simulink model "car_model_FIXED"  (R2022b)
settings: Solver=VariableStepAuto  StartTime=0.0  StopTime=60  RelTol=1e-3
values from neighbouring files (symbols this model uses):
  ABS_MAX_TORQUE = [25 25 25 25]    [Startup.m]
  ABS_MAX_TRQ_CMD = dot(ABS_MAX_TORQUE, MOTOR_ENABLE)    [Startup.m]
  ABS_MIN_TORQUE = [0.01 0.01 0.01 0.01]    [Startup.m]
  acc_IC = 0    [Startup.m]
  ACCELERATION_MAX = 30    [Startup.m]
  ang_IC = 0    [Startup.m]
  ang_vel_IC = 0    [Startup.m]
  ax = Reference_Signals.Chassis_Acceleration_VNED.ax.Data(:)    [Simulation_Data_Parse.m]    (also in Vehicle_Sim_Parse.m)
  ay = Reference_Signals.Chassis_Acceleration_VNED.ay.Data(:)    [Simulation_Data_Parse.m]    (also in Vehicle_Sim_Parse.m)
  az = Reference_Signals.Chassis_Acceleration_VNED.az.Data(:)    [Simulation_Data_Parse.m]    (also in Vehicle_Sim_Parse.m)
  battery_current_IC = 0    [Startup.m]
  BATTERY_CURRENT_MAX = 140    [Startup.m]
  BATTERY_CURRENT_MIN = 0    [Startup.m]
  battery_FT_IC = 300    [Startup.m]
  battery_T_IC = 300    [Startup.m]
  BATTERY_TEMPERATURE_MAX = 60    [Startup.m]
  BATTERY_TEMPERATURE_MIN = 0    [Startup.m]
  battery_voltage_IC = Ns*max(Em)    [Startup.m]
  BATTERY_VOLTAGE_MAX = 340    [Startup.m]
  BATTERY_VOLTAGE_MIN = 60    [Startup.m]
  Brake_Pressure_IC = 1    [Startup.m]
  ccl_IC = 0    [Startup.m]
  CENTER_STEER_ANGLE_MAX = 130    [Startup.m]
  covarience_matrix_IC = Simulink.Parameter(eye(28)./1000)    [Startup.m]
  dcl_IC = 140    [Startup.m]
  DCL_MAX = 130    [Startup.m]
  DCL_MIN = 0    [Startup.m]
  driver_t = 0.015    [Startup.m]
  fusion_t = Simulink.Parameter(0.01)    [Startup.m]
  fusion_t_sim = fusion_t.copy    [Startup.m]
  Fz_IC = m_all*g/4    [Startup.m]
  g = 9.81    [Startup.m]
  gps_hz = 0.01    [Startup.m]
  gps_ratio = Simulink.Parameter(gps_hz / imu_hz.Value)    [Startup.m]
  imu_hz = fusion_t.copy    [Startup.m]
  location_lla_IC = Simulink.Parameter([40.437675, -86.943750, 200])    [Startup.m]
  MAG_MAX = 200    [Startup.m]
  Max_Brake_Pressure = 10^8    (= 100000000)    [Startup.m]
  Max_Driver_Input = 1    [Startup.m]
  MAX_DTHETA_DRIVER = 360    [Startup.m]
  MAX_STEERING_ADJUST = 15    [Startup.m]
  Min_Brake_Pressure = 1    [Startup.m]
  Min_Driver_Input = 0    [Startup.m]
  motor_current_IC = 0    [Startup.m]
  MOTOR_CURRENT_MAX = 70    [Startup.m]
  MOTOR_CURRENT_MIN = 0    [Startup.m]
  MOTOR_ENABLE = [0 0 1 1]    [Startup.m]
  motor_FT_IC = 300    [Startup.m]
  motor_T_IC = 300    [Startup.m]
  MOTOR_TEMPERATURE_MAX = 100    [Startup.m]
  MOTOR_TEMPERATURE_MIN = 0    [Startup.m]
  motor_voltage_IC = 332    [Startup.m]
  MOTOR_VOLTAGE_MAX = 340    [Startup.m]
  MOTOR_VOLTAGE_MIN = 90    [Startup.m]
  omega_IC = 0    [Startup.m]
  OMEGA_MAX = 150    [Startup.m]
  OMEGA_MIN = 0    [Startup.m]
  ORIENTATION_MAX = 360    [Startup.m]
  pos_IC = 0    [Startup.m]
  POS_MAX = 300    [Startup.m]
  rho = 1.225    [Startup.m]
  selected_maxvm = MIN_TRACK_DATA.(event_names(10))    [Startup.m]
  selected_sweep = ALL_SWEEP_DATA.(sweep_names(1))    [Startup.m]
  selected_track = ALL_TRACK_DATA.(event_names(10))    [Startup.m]
  shock_length_IC = 0.1    [Startup.m]
  SHOCK_LENGTH_MAX = 0.25    [Startup.m]
  SHOCK_LENGTH_MIN = 0    [Startup.m]
  state_IC = zeros(28,1)    [Startup.m]
  theta_IC = 0    [Startup.m]
  TRACTION_ENABLE = 0    [Startup.m]
  TVS_ENABLE = 0    [Startup.m]
  tvs_t = 0.015    [Startup.m]
  tvs_t_sim = tvs_t    (= 0.015)    [Startup.m]
  Tx_I = 0    [Startup.m]
  vel_IC = [0 0 0]    [Startup.m]
  VELOCITY_MAX = 30    [Startup.m]
  X = Reference_Signals.Chassis_Position.X.Data(:)    [Simulation_Data_Parse.m]    (also in Vehicle_Sim_Parse.m = Chassis_Signals.InertFrm.Cg.Disp.X.Data(:))
  Y = Reference_Signals.Chassis_Position.Y.Data(:)    [Simulation_Data_Parse.m]    (also in Vehicle_Sim_Parse.m = Chassis_Signals.InertFrm.Cg.Disp.Y.Data(:))
  YAW_ENABLE = 1    [Startup.m]
  YAW_MAX = 2.5    [Startup.m]
undefined symbols (not defined in the file or in its folder): ActSuspDutyCycle, Aeq_left, Aeq_right, alpha_error, ang_acc_hystersesis, area_air, axb, br, brake_bias, covA, covG, covM, covP, covV, CURRENT_BUFFER, cy_sweep, dB, deadband_angle, dIndex, DiscIntNeverNeededParam, dt_OFF, dt_ON, dTx, dx, dZ, efficiency_grid, F0z, forward_look_straight, forward_look_turn, Fz_sweep, GAIN_ABS, gearbox_efficiency, gr, I, I_Driver, IMU_accel, IMU_gyro, IMU_mag, IMUNED2VNED, indicies, IYY, kx_sweep, l, lambda_star, low_V_SA, lr, m_all, m_body, m_unsprung, MAGNED2VNED, MAX_I_Driver, max_yaw, min_velocity_regen, motorControllerCurve, motorTempCurve, motorTempX, mu_star, mx_sweep, my_sweep, noise_state ... (+40)
libraries: fl_lib x82, nesl_utility x32, vehdynlibtire x10, vehdynlibsuspension x8, simulink x5, autolibutils x5, sharedtransform x5, sdl_lib x4, EngineCoolingComponents_lib x4, slpidlib x3, SimscapeFluids_lib x3, shared6dof x2
(part 4 of 14)

== system car_model_FIXED/Vehicle Model/Suspension ==
  Steering : Inport
  Wheel : Inport  Port=2
  Vehicle : Inport  Port=3
  Double Wishbone Suspension : Subsystem  VariantControl=1
      mask Display: image('suspdw.png');
  Independent Mapped Front Suspension Mapped Solid Axle Rear Suspension : Subsystem  VariantControl=2
      mask Display: image([imread('suspindmap.png');imread('suspsamap.png')]);
  Kinematics and Compliance Independent Suspension : Subsystem  VariantControl=6
      mask Display: image('suspkandc.png');
  MacPherson Front Suspension Solid Axle Rear Suspension : Subsystem  VariantControl=3
      mask Display: image([imread('suspmacp.png');imread('suspsacoil.png')]);
  MacPherson Suspension : Subsystem  VariantControl=4
      mask Display: image('suspmacp.png');
  Mapped Suspension : Subsystem  VariantControl=5
      mask Display: image('suspindmap.png');
  Suspension : Outport  VectorParamsAs1DForOutWhenUnconnected=off
  Suspension1 : Outport  Port=2  VectorParamsAs1DForOutWhenUnconnected=off
  Veh : Outport  Port=3  VectorParamsAs1DForOutWhenUnconnected=off

== system car_model_FIXED/Vehicle Model/Vehicle ==
  Suspension : Inport
  6DOF : Subsystem  VariantControl=1
  Constant : Constant  Value=[0 0 0]
  VehFdbk : Outport  VectorParamsAs1DForOutWhenUnconnected=off
  wires:
  6DOF/1(VehFdbk) -> VehFdbk/1  "VehFdbk"
  Constant/1 -> 6DOF/2(Wind)
  Suspension/1 -> 6DOF/1(Suspension)

== system car_model_FIXED/Vehicle Model/Wheels and Tires ==
  Brake Press : Inport  Unit=Pa
  PwrTrn : Inport  Port=2
  Sus : Inport  Port=3
  Veh : Inport  Port=4
  Bus Selector : BusSelector  OutputSignals=axle_torque
  Bus Selector1 : BusSelector  OutputSignals=Whl.Ang,Whl.F,Whl.AngVel,Whl.xdot,Whl.ydot
  Bus Selector2 : BusSelector  OutputSignals=BdyFrm.Cg.Vel.xdot,BdyFrm.Cg.Vel.ydot  OutputAsBus=on
  Constant1 : Constant  Value=[1 1 1 1].*0.00182
  Constant3 : Constant  Value=[1 1 1 1]
  Cont LPF : autolibutils/Cont LPF  wc=100*2*pi  AbsoluteTolerance=auto  aMode=2
  Cont LPF1 : autolibutils/Cont LPF  wc=100*2*pi  AbsoluteTolerance=auto  aMode=2
  Matrix Concatenate : Concatenate  NumInputs=3  Mode=Multidimensional array
  Reshape{1..4} (4 alike) : Reshape
  Saturation : Saturate  UpperLimit=inf  LowerLimit=-10*9.81*2000  ZeroCross=off
  Selector : Selector  NumberOfDimensions=2  InputPortWidth=3  IndexOptions=Index vector (dialog),Select all  Indices=[3],1  OutputSizes=1,1
  Selector1 : Selector  NumberOfDimensions=2  InputPortWidth=1  IndexOptions=Index vector (dialog),Select all  Indices=[3],1  OutputSizes=1,1
  Selector2 : Selector  NumberOfDimensions=2  InputPortWidth=3  IndexOptions=Index vector (dialog),Select all  Indices=3,1  OutputSizes=1,1
  Selector3 : Selector  NumberOfDimensions=2  InputPortWidth=3  IndexOptions=Index vector (dialog),Select all  Indices=1,1  OutputSizes=1,1
  Sqrt : Sqrt
  Square : Math  Operator=square
  Sum : Sum  Inputs=+
  Terminator{,1..2,4..5} (5 alike) : Terminator
  VDBS : Subsystem  VariantControl=0
  Vehicle : Outport  VectorParamsAs1DForOutWhenUnconnected=off
  Suspension : Outport  Port=2  VectorParamsAs1DForOutWhenUnconnected=off
  Wheels : Outport  Port=3  VectorParamsAs1DForOutWhenUnconnected=off
  Power Train : Outport  Port=4  VectorParamsAs1DForOutWhenUnconnected=off
  Wheels2Susp : Outport  Port=5  VectorParamsAs1DForOutWhenUnconnected=off
  Vg : Outport  Port=6  VectorParamsAs1DForOutWhenUnconnected=off
  wires:
  Bus Selector1/2 -> Selector/1  "<F>"
  VDBS/3(FrntAxlF) -> Terminator/1
  VDBS/4(RearAxlF) -> Terminator1/1
  VDBS/6(Mz) -> Terminator4/1
  Selector1/1 -> Reshape1/1
  Matrix Concatenate/1 -> VDBS/7(VehVel)
  PwrTrn/1 -> Power Train/1, Bus Selector/1
  Reshape4/1 -> VDBS/1(WhlAng)  "WhlAng"
  Reshape3/1 -> VDBS/2(WhlCmb)  "WhlCmb"
  Selector/1 -> Reshape2/1
  Saturation/1 -> VDBS/5(Fz)
  Constant1/1 -> VDBS/8(Ground Level)
  VDBS/8(SuspWhlVz) -> Matrix Concatenate/3  "zdot"
  Bus Selector1/1 -> Cont LPF1/1  "<Ang>"
  Selector3/1 -> Reshape3/1  "Camber Angles"
  Sus/1 -> Suspension/1, Bus Selector1/1
  Bus Selector1/4 -> Matrix Concatenate/1  "<xdot>"
  Bus Selector1/5 -> Matrix Concatenate/2  "<ydot>"
  VDBS/7(SuspWhlPz) -> Terminator5/1  "z"
  Reshape2/1 -> Cont LPF/1
  Bus Selector1/3 -> Selector1/1  "<AngVel>"
  Reshape1/1 -> VDBS/6(r)
  Brake Press/1 -> VDBS/4(BrkPed)
  Constant3/1 -> VDBS/9(Friction)
  Cont LPF/1 -> Saturation/1
  Cont LPF1/1 -> Selector3/1, Selector2/1
  Selector2/1 -> Reshape4/1  "Wheel Angles"
  Veh/1 -> Vehicle/1, Bus Selector2/1, VDBS/10(Veh)  "Veh"
  VDBS/2(Wheels2Susp) -> Wheels2Susp/1  "Wheels"
  VDBS/1(Wheels) -> Wheels/1
  Bus Selector/1 -> VDBS/3(AxleTrq)  "<axle_torque>"
  VDBS/5(Omega) -> Terminator2/1
  Bus Selector2/1 -> Square/1
  Square/1 -> Sum/1
  Sum/1 -> Sqrt/1
  Sqrt/1 -> Vg/1

== system car_model_FIXED/Control Systems/CLC/Step ==
  DTC_output_1 : DataTypeConversion  OutDataTypeStr=fixdt('double')  SaturateOnIntegerOverflow=off  RndMeth=Floor
  ReplicaOfSource : Step  After=0  SampleTime=0
  Out1 : Outport  LockScale=on
  wires:
  DTC_output_1/1 -> Out1/1
  ReplicaOfSource/1 -> DTC_output_1/1

== system car_model_FIXED/Control Systems/Sensor Fusion/Coordinate Back Transform ==
  rot_map : Inport  OutMin=-1  OutMax=1  OutDataTypeStr=fixdt(1,32,30)
  vel_NED : Inport  Port=2  OutMin=-VELOCITY_MAX  OutMax=VELOCITY_MAX  OutDataTypeStr=fixdt(1,32,26)
  accel_NED : Inport  Port=3  OutMin=-ACCELERATION_MAX  OutMax=ACCELERATION_MAX  OutDataTypeStr=fixdt(1,32,26)
  accel_bias_NED : Inport  Port=4  OutMin=-ACCELERATION_MAX  OutMax=ACCELERATION_MAX  OutDataTypeStr=fixdt(1,32,26)
  gyro_bias_NED : Inport  Port=5  OutMin=-YAW_MAX  OutMax=YAW_MAX  OutDataTypeStr=fixdt(1,32,29)
  Product : Product  Multiplication=Matrix(*)  OutDataTypeStr=fixdt(1,32,24)
  Product1 : Product  Multiplication=Matrix(*)  OutDataTypeStr=fixdt(1,32,24)
  Product2 : Product  Multiplication=Matrix(*)  OutDataTypeStr=fixdt(1,32,24)
  Product3 : Product  Multiplication=Matrix(*)  OutDataTypeStr=fixdt(1,32,28)
  vel_VNED : Outport  OutMin=-VELOCITY_MAX  OutMax=VELOCITY_MAX
  acc_VNED : Outport  Port=2  OutMin=-ACCELERATION_MAX  OutMax=ACCELERATION_MAX
  acc_bias_VNED : Outport  Port=3  OutMin=-ACCELERATION_MAX  OutMax=ACCELERATION_MAX
  gyro_bias_VNED : Outport  Port=4  OutMin=-YAW_MAX  OutMax=YAW_MAX
  wires:
  gyro_bias_NED/1 -> Product3/2
  vel_NED/1 -> Product/2
  Product2/1 -> acc_bias_VNED/1  "acc_bias_VNED"
  Product1/1 -> acc_VNED/1  "acc_VNED"
  rot_map/1 -> Product3/1, Product2/1, Product1/1, Product/1
  Product/1 -> vel_VNED/1  "vel_VNED"
  Product3/1 -> gyro_bias_VNED/1  "gyro_bias_VNED"
  accel_bias_NED/1 -> Product2/2
  accel_NED/1 -> Product1/2

== system car_model_FIXED/Control Systems/Sensor Fusion/Coordinate Transformation ==
  accel : Inport  OutMin=-ACCELERATION_MAX  OutMax=ACCELERATION_MAX  OutDataTypeStr=fixdt(1,32,26)  PortDimensions=[3 1]
  gyro : Inport  Port=2  OutMin=-YAW_MAX  OutMax=YAW_MAX  OutDataTypeStr=fixdt(1,32,29)  PortDimensions=[3 1]
  mag : Inport  Port=3  OutMin=-MAG_MAX  OutMax=MAG_MAX  OutDataTypeStr=fixdt(1,32,23)  PortDimensions=[3 1]
  Constant : Constant  Value=IMUNED2VNED  OutDataTypeStr=fixdt(1,32,30)
  Constant1 : Constant  Value=MAGNED2VNED  OutDataTypeStr=fixdt(1,32,31)
  Product : Product  Multiplication=Matrix(*)  OutDataTypeStr=fixdt(1,32,24)
  Product1 : Product  Multiplication=Matrix(*)  OutDataTypeStr=fixdt(1,32,21)
  Product2 : Product  Multiplication=Matrix(*)  OutDataTypeStr=fixdt(1,32,28)
  acc_VNED : Outport  OutMin=-ACCELERATION_MAX  OutMax=ACCELERATION_MAX  PortDimensions=[3 1]
  angvel_VNED : Outport  Port=2  OutMin=-YAW_MAX  OutMax=YAW_MAX  PortDimensions=[3 1]
  mag_VNED : Outport  Port=3  OutMin=-MAG_MAX  OutMax=MAG_MAX  PortDimensions=[3 1]
  wires:
  Product/1 -> acc_VNED/1  "accel_VNED"
  accel/1 -> Product/2
  Product2/1 -> angvel_VNED/1  "gyro_VNED"
  Constant1/1 -> Product1/1
  mag/1 -> Product1/2
  Product1/1 -> mag_VNED/1  "mag_VNED"
  gyro/1 -> Product2/2
  Constant/1 -> Product2/1, Product/1

== system car_model_FIXED/Control Systems/Sensor Fusion/SFS ==
  velocity : Inport  OutMin=-VELOCITY_MAX  OutMax=VELOCITY_MAX  OutDataTypeStr=double
  position : Inport  Port=2  OutMin=-POS_MAX  OutMax=POS_MAX  OutDataTypeStr=double
  acceleration : Inport  Port=3  OutMin=-ACCELERATION_MAX  OutMax=ACCELERATION_MAX  OutDataTypeStr=double  PortDimensions=[3 1]
  angularVelocity : Inport  Port=4  OutMin=-YAW_MAX  OutMax=YAW_MAX  OutDataTypeStr=double  PortDimensions=[3 1]
  mag : Inport  Port=5  OutMin=-MAG_MAX  OutMax=MAG_MAX  OutDataTypeStr=double  PortDimensions=[3 1]
  Unit Delay2 : UnitDelay  InitialCondition=state_IC  SampleTime=-1  HasFrameUpgradeWarning=on
  Unit Delay3 : UnitDelay  InitialCondition=covarience_matrix_IC  SampleTime=-1  HasFrameUpgradeWarning=on
  fusion : MATLAB Function  TreatAsAtomicUnit=on
  ang_VNED : Outport  OutMin=-1  OutMax=1  OutDataTypeStr=double
  angvel_VNED : Outport  Port=2  OutMin=-YAW_MAX  OutMax=YAW_MAX  OutDataTypeStr=double
  pos_VNED : Outport  Port=3  OutMin=-POS_MAX  OutMax=POS_MAX  OutDataTypeStr=double
  mag_NED : Outport  Port=4  OutMin=-MAG_MAX  OutMax=MAG_MAX  OutDataTypeStr=double
  mag_bias_VNED : Outport  Port=5  OutMin=-MAG_MAX  OutMax=MAG_MAX  OutDataTypeStr=double
  rot_map : Outport  Port=6  OutMin=-1  OutMax=1  OutDataTypeStr=double
  vel_NED : Outport  Port=7  OutMin=-VELOCITY_MAX  OutMax=VELOCITY_MAX  OutDataTypeStr=double
  accel_NED : Outport  Port=8  OutMin=-ACCELERATION_MAX  OutMax=ACCELERATION_MAX  OutDataTypeStr=double
  accel_bias_NED : Outport  Port=9  OutMin=-ACCELERATION_MAX  OutMax=ACCELERATION_MAX  OutDataTypeStr=double
  gyro_bias_NED : Outport  Port=10  OutMin=-YAW_MAX  OutMax=YAW_MAX  OutDataTypeStr=double
  wires:
  angularVelocity/1 -> fusion/5(angularVelocity)
  fusion/12(cov_out) -> Unit Delay3/1
  Unit Delay3/1 -> fusion/7(cov_in)
  position/1 -> fusion/3(position)
  acceleration/1 -> fusion/4(acceleration)
  velocity/1 -> fusion/2(velocity)
  fusion/2(rot_map) -> rot_map/1
  mag/1 -> fusion/6(magField)
  fusion/1(state_out) -> Unit Delay2/1
  Unit Delay2/1 -> fusion/1(state_in)
  fusion/3(ang) -> ang_VNED/1
  fusion/4(angvel) -> angvel_VNED/1
  fusion/5(pos) -> pos_VNED/1
  fusion/6(vel) -> vel_NED/1
  fusion/7(accel) -> accel_NED/1
  fusion/8(mag) -> mag_NED/1
  fusion/9(accel_bias) -> accel_bias_NED/1
  fusion/10(gyro_bias) -> gyro_bias_NED/1
  fusion/11(mag_bias) -> mag_bias_VNED/1

== system car_model_FIXED/Control Systems/TVS/Optimization ==
  note: reduce this limit?
  driver_input : Inport  OutDataTypeStr=double
  obj_gain : Inport  Port=2
  b : Inport  Port=3  OutDataTypeStr=double
  ub : Inport  Port=4  OutDataTypeStr=double
  lb : Inport  Port=5  OutDataTypeStr=double
  Aeq : Inport  Port=6  OutDataTypeStr=double
  beq : Inport  Port=7  OutDataTypeStr=double
  A Dot : DotProduct  OutDataTypeStr=double
  Aeq Dot : DotProduct  OutDataTypeStr=double
  C Caller : CCaller  FunctionName=bigM_func  PortSpecificationStruct="%)30     .    N\"X   8    (     @         %    \"    !P    !     0         %  0 \"0    $    _    07)G3F%M90  4&]R=$YA;64 4V-O<&4     26YD97@     5'EP90      4VEZ90      27-';&]B86P   X    P    !@    @    $          4    (     0    ,    !         !   P!O=70 #@   #     &    \"     0         !0    @    !     P    $         $  # &]U=  .    .     8    (    !          %    \"     $    &     0         0  ...(+15750 chars)"
  Constant : Constant  Value=TVS_ENABLE
  Constant1 : Constant  Value=[1 1 1 1]
  Demux{,1..4} (5 alike) : Demux
  Switch : Switch  Criteria=u2 > Threshold  SaturateOnIntegerOverflow=off  InputSameDT=off
  Tx_RAW_demux : Mux
  Tx_choose : Switch  Criteria=u2 > Threshold  Threshold=2  OutDataTypeStr=double  SaturateOnIntegerOverflow=off  InputSameDT=off
  Tx_deadband : DeadZone  LowerValue=-10*dTx  UpperValue=10*dTx  SaturateOnIntegerOverflow=off
  Tx_equal_gain : Gain  Gain=ABS_MAX_TORQUE.*MOTOR_ENABLE  OutDataTypeStr=double
  Tx_equal_offset : Bias  Bias=ABS_MAX_TORQUE  SaturateOnIntegerOverflow=off
  Tx_initial : Constant  Value=Tx_I  OutDataTypeStr=double
  Tx_rate_limit : RateLimiter  RisingSlewLimit=Torque_Up_Rate_Limit  FallingSlewLimit=-Torque_Down_Rate_Limit  SampleTimeMode=inherited
  Tx_reverse_offset : Bias  Bias=-ABS_MAX_TORQUE  SaturateOnIntegerOverflow=off
  b Add : Sum  OutDataTypeStr=double
  beq Add : Sum  OutDataTypeStr=double
  lb_offset : Bias  Bias=ABS_MAX_TORQUE  SaturateOnIntegerOverflow=off
  optimization_offset_A : Constant  Value=ABS_MAX_TORQUE  OutDataTypeStr=double
  optimization_offset_Aeq : Constant  Value=ABS_MAX_TORQUE  OutDataTypeStr=double
  ub_offset : Bias  Bias=ABS_MAX_TORQUE  SaturateOnIntegerOverflow=off
  yaw_error_limit : Constant  Value=yaw_error_limit  OutDataTypeStr=double
  Tx : Outport
  exitflag : Outport  Port=2
  wires:
  C Caller/1 -> Tx_choose/2, exitflag/1  "exitflag"
  lb/1 -> lb_offset/1  "lb"
  ub/1 -> ub_offset/1  "ub"
  C Caller/2 -> Tx_RAW_demux/1  "TFL"
  C Caller/5 -> Tx_RAW_demux/4  "TRR"
  C Caller/4 -> Tx_RAW_demux/3  "TRL"
  C Caller/3 -> Tx_RAW_demux/2  "TFR"
  Demux/1 -> C Caller/1  "obj_FL"
  Demux/2 -> C Caller/2  "obj_FR"
  Demux/3 -> C Caller/3  "obj_RL"
  Demux/4 -> C Caller/4  "obj_RR"
  Tx_initial/1 -> C Caller/23, C Caller/24, C Caller/26, C Caller/25  "Tx_initial"
  Demux1/1 -> C Caller/19  "ub_FL"
  Demux1/2 -> C Caller/20  "ub_FR"
  Demux1/3 -> C Caller/21  "ub_RL"
  Demux1/4 -> C Caller/22  "ub_RR"
  Demux2/1 -> C Caller/15  "lb_FL"
  Demux2/2 -> C Caller/16  "lb_FR"
  Demux2/3 -> C Caller/17  "lb_RL"
  Demux2/4 -> C Caller/18  "lb_RR"
  Demux3/3 -> C Caller/13  "Aeq_RL"
  Demux3/2 -> C Caller/12  "Aeq_FR"
  Demux3/1 -> C Caller/11  "Aeq_FL"
  Demux3/4 -> C Caller/14  "Aeq_RR"
  Demux4/1 -> C Caller/6  "A_FL"
  Demux4/2 -> C Caller/7  "A_FR"
  Demux4/3 -> C Caller/8  "A_RL"
  Demux4/4 -> C Caller/9  "A_RR"
  ub_offset/1 -> Demux1/1  "ub_b"
  optimization_offset_Aeq/1 -> Aeq Dot/1  "offset"
  optimization_offset_A/1 -> A Dot/1  "offset"
  beq/1 -> beq Add/1  "beq"
  Aeq Dot/1 -> beq Add/2  "Aeq_b"
  b/1 -> b Add/1  "b"
  A Dot/1 -> b Add/2
  yaw_error_limit/1 -> C Caller/27  "yaw_error_limit"
  Tx_RAW_demux/1 -> Tx_choose/1  "Tx_RAW_TV"
  Constant1/1 -> Demux4/1, A Dot/2  "A"
  b Add/1 -> C Caller/5  "b_b"
  obj_gain/1 -> Demux/1  "obj_gain"
  lb_offset/1 -> Demux2/1  "lb_b"
  Aeq/1 -> Demux3/1, Aeq Dot/2  "Aeq"
  beq Add/1 -> C Caller/10  "beq_b"
  Tx_rate_limit/1 -> Tx/1  "Tx"
  Tx_reverse_offset/1 -> Tx_deadband/1
  driver_input/1 -> Tx_equal_gain/1
  Tx_deadband/1 -> Tx_rate_limit/1
  Tx_choose/1 -> Switch/1
  Tx_equal_gain/1 -> Tx_equal_offset/1  "Tx_equal"
  Tx_equal_offset/1 -> Switch/3, Tx_choose/3
  Switch/1 -> Tx_reverse_offset/1
  Constant/1 -> Switch/2

== system car_model_FIXED/Control Systems/TVS/Power Controller ==
  note: Tune the distance before PL is enabled
  note: Create a better map wherein you have T,V,I,w
  note: Tune the endpoints
  vel : Inport  OutDataTypeStr=double
  battery_voltage : Inport  Port=2
  pack_current : Inport  Port=3
  dcl : Inport  Port=4  OutDataTypeStr=double  LockScale=on
  ccl : Inport  Port=5  OutDataTypeStr=double  LockScale=on
  driver_input : Inport  Port=6  OutDataTypeStr=double  LockScale=on
  motor_temp : Inport  Port=7
  mc_temp : Inport  Port=8
  omega : Inport  Port=9
  Abs Max Torque CMD (Nm) : Constant  Value=ABS_MAX_TRQ_CMD
  Constant2 : Constant  Value=[0 0 0 0]  OutDataTypeStr=double
  Constant3 : Constant  Value=ABS_MAX_TORQUE
  Current to Torque : Gain  Gain=ABS_MAX_TRQ_CMD/BATTERY_CURRENT_MAX
  Gain4 : Gain  Gain=-MOTOR_ENABLE  ParamDataTypeStr=double  OutDataTypeStr=Inherit: Inherit via back propagation
  Gain8 : Gain  Gain=MOTOR_ENABLE  ParamDataTypeStr=double  OutDataTypeStr=Inherit: Inherit via back propagation
  Max : MinMax  Function=max
  Max Torque : Saturate  UpperLimit=ABS_MAX_TORQUE  LowerLimit=dTx  OutDataTypeStr=Inherit: Inherit via back propagation
  Max Torque Command Selector : Switch  Criteria=u2 > Threshold  Threshold=CURRENT_BUFFER  SaturateOnIntegerOverflow=off  InputSameDT=off
  Max1 : MinMax  Function=max
  Min Throttle Command (Nm) : Constant  Value=dTx*10
  Min Torque : Saturate  UpperLimit=ABS_MIN_TORQUE  LowerLimit=0  OutDataTypeStr=Inherit: Inherit via back propagation
  Minimum : MinMax  Inputs=3
  Selector : Selector  InputPortWidth=4  IndexOptions=Index vector (dialog)  Indices=4  OutputSizes=1
  Subtract : Sum  Inputs=+-
  Switch1 : Switch  Threshold=min_velocity_regen  OutDataTypeStr=Inherit: Inherit via back propagation  SaturateOnIntegerOverflow=off  InputSameDT=off
  Temperature to Motor Controller Current Limit Map : Lookup_n-D  NumberOfTableDimensions=1  BreakpointsForDimension1=motorControllerCurve(:,1)  IndexSearchMethod=Evenly spaced points  Table=motorControllerCurve(:,2)  ExtrapMethod=Clip  UseLastTableValue=on  InternalRulePriority=Speed  RndMeth=Simplest
  Temperature to Motor Current Limit Map : Lookup_n-D  NumberOfTableDimensions=1  BreakpointsForDimension1=motorTempX  IndexSearchMethod=Evenly spaced points  Table=motorTempCurve  ExtrapMethod=Clip  UseLastTableValue=on  InternalRulePriority=Speed  RndMeth=Simplest
  Terminator : Terminator
  Terminator1 : Terminator
  Terminator2 : Terminator
  "Throttle Map " : Subsystem  Tag=DecoupledSystem
  Throttle Saturation : simulink/Discontinuities/Saturation Dynamic  OutMin=[0]  OutMax=[]  OutDataTypeStr=Inherit: Same as second input  OutDataType=fixdt(1, 16)  OutScaling=2^-10  DoSatur=off
  Throttle to Torque : Gain  Gain=ABS_MAX_TRQ_CMD
  b : Outport  OutDataTypeStr=double  LockScale=on
  Max b : Outport  Port=2  OutDataTypeStr=double  LockScale=on
  ub : Outport  Port=3  OutDataTypeStr=double  LockScale=on
  lb : Outport  Port=4  OutDataTypeStr=double  LockScale=on
  wires:
  Max1/1 -> Temperature to Motor Controller Current Limit Map/1
  Temperature to Motor Current Limit Map/1 -> Minimum/2  "Total Motor Current Limit (A)"
  battery_voltage/1 -> Terminator1/1
  Min Throttle Command (Nm)/1 -> Throttle Saturation/3
  Gain8/1 -> Max Torque/1
  Constant3/1 -> Gain4/1, Gain8/1
  Throttle Saturation/1 -> b/1  "Limited Torque CMD (Nm)"
  Max/1 -> Temperature to Motor Current Limit Map/1
  Gain4/1 -> Min Torque/1
  Constant2/1 -> Switch1/3  "Abs Min Torque CMD"
  Selector/1 -> Switch1/2  "Planer Vcog (m/s)"
  motor_temp/1 -> Max/1  "[FL FR RL RR] Motor Temperature (degC)"
  ccl/1 -> Terminator/1
  driver_input/1 -> "Throttle Map "/1(In1)  "RAW Throttle"
  Max Torque/1 -> ub/1  "Max Individual Motor Torque (Nm)"
  "Throttle Map "/1(Out1) -> Throttle to Torque/1  "Mapped Throttle"
  Throttle to Torque/1 -> Throttle Saturation/2  "RAW Torque CMD (Nm)"
  mc_temp/1 -> Max1/1  "[FL FR RL RR] Motor Controller Temperature (degC)"
  dcl/1 -> Minimum/1  "Discharge Current Limit (A)"
  vel/1 -> Selector/1  "[Vx Vy Vcog]"
  Temperature to Motor Controller Current Limit Map/1 -> Minimum/3  "Total Motor Controller Current Limit (A)"
  Min Torque/1 -> Switch1/1
  Switch1/1 -> lb/1  "Min Individual Motor Torque (Nm)"
  Subtract/1 -> Max Torque Command Selector/2  "Distance to DCL (A)"
  Abs Max Torque CMD (Nm)/1 -> Max Torque Command Selector/1
  Current to Torque/1 -> Max Torque Command Selector/3  "Temperature Dependent Max Torque CMD (Nm)"
  pack_current/1 -> Subtract/2  "pack_current (A)"
  Minimum/1 -> Current to Torque/1, Subtract/1  "Max Allowed Pack Current (A)"
  Max Torque Command Selector/1 -> Max b/1, Throttle Saturation/1  "Max Allowed Torque CMD (Nm)"
  omega/1 -> Terminator2/1

== system car_model_FIXED/Control Systems/TVS/Traction Controller ==
  Fz : Inport  OutDataTypeStr=double  LockScale=on
  vel : Inport  Port=2  OutDataTypeStr=double  LockScale=on
  ang_vel : Inport  Port=3  OutDataTypeStr=double  LockScale=on
  CCSA : Inport  Port=4
  omega : Inport  Port=5
  1-D Lookup Table : Subsystem  Tag=DecoupledSystem
  1-D Lookup Table1 : Subsystem  Tag=DecoupledSystem
  1-D Lookup Table2 : Subsystem  Tag=DecoupledSystem
  1-D Lookup Table3 : Subsystem  Tag=DecoupledSystem
  Compute SA : Subsystem
  Compute SL : Subsystem
  Compute SL Fake : Subsystem
  Constant : Constant
  Constant1 : Constant  Value=[1 1 1 1].*low_V_SA
  Constant2 : Constant  Value=TRACTION_ENABLE
  Divide : Product  Inputs=**//
  Divide1 : Product  Inputs=**//
  Gain : Gain  Gain=gr./RE
  Selector : Selector  InputPortWidth=4  IndexOptions=Index vector (dialog)  Indices=4  OutputSizes=1
  Selector1 : Selector  InputPortWidth=4  IndexOptions=Index vector (dialog)  Indices=4  OutputSizes=1
  Sqrt : Sqrt
  Square : Math  Operator=square
  Square1 : Math  Operator=square
  Steering Model : Subsystem
  Sum : Sum  Inputs=|++
  Switch : Switch  Criteria=u2 > Threshold  Threshold=Vth  SaturateOnIntegerOverflow=off  InputSameDT=off
  Switch1 : Switch  Criteria=u2 > Threshold  Threshold=Vth  SaturateOnIntegerOverflow=off  InputSameDT=off
  Switch2 : Switch  Criteria=u2 > Threshold  SaturateOnIntegerOverflow=off  InputSameDT=off
  obj_gain : Outport
  wires:
  Gain/1 -> obj_gain/1  "obj_gain"
  Constant/1 -> Gain/1, Switch2/3
  Sum/1 -> Sqrt/1
  Divide/1 -> Square/1  "a_bar"
  1-D Lookup Table/1(Out1) -> Divide/2
  1-D Lookup Table1/1(Out1) -> Divide/3
  Fz/1 -> 1-D Lookup Table1/1(In1), Divide/4, 1-D Lookup Table2/1(In1), 1-D Lookup Table3/1(In1), Divide1/4, 1-D Lookup Table/1(In1)
  Divide1/1 -> Square1/1  "s_bar"
  1-D Lookup Table2/1(Out1) -> Divide1/2
  1-D Lookup Table3/1(Out1) -> Divide1/3
  Switch/1 -> Divide1/1
  Switch1/1 -> Divide/1
  Compute SL Fake/1(SL_fake) -> Switch/3
  Compute SL/1(Out1) -> Switch/1
  Compute SA/1(Out1) -> Switch1/1, Compute SL/1(In1)
  vel/1 -> Compute SL/3(Vg), Selector/1, Compute SL Fake/2(Vg), Selector1/1, Compute SA/3(Vg)
  ang_vel/1 -> Compute SA/2(ang_vel)
  omega/1 -> Compute SL Fake/1(omega), Compute SL/2(omega)
  Steering Model/1(steering) -> Compute SA/1(steering)
  Constant1/1 -> Switch1/3
  Sqrt/1 -> Switch2/1
  Constant2/1 -> Switch2/2
  Selector/1 -> Switch/2
  Selector1/1 -> Switch1/2
  Square/1 -> Sum/1
  Square1/1 -> Sum/2
  CCSA/1 -> Steering Model/1(steering_angle)
